simulink model "gm_sampleModel2076_4_sub"  (R2023a)
settings: Solver=VariableStepAuto  StartTime=0.0  StopTime=10.0  RelTol=1e-3
libraries: hdlsllib x2, simulink x1
settings Model: Creator=user1  LastModifiedBy=user1
settings OptimizationCC: BlockReduction=off  ConditionallyExecuteInputs=off
settings DebuggingCC: InheritedTsInSrcMsg=none

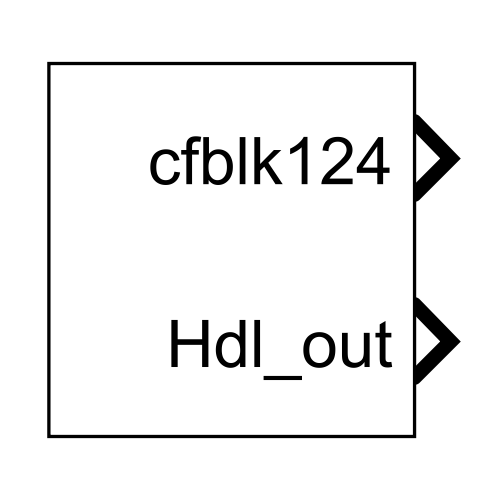
[thumbnail: Simulink's stored preview of the top-level diagram]
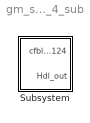
== system gm_sampleModel2076_4_sub ==
  Subsystem : Subsystem

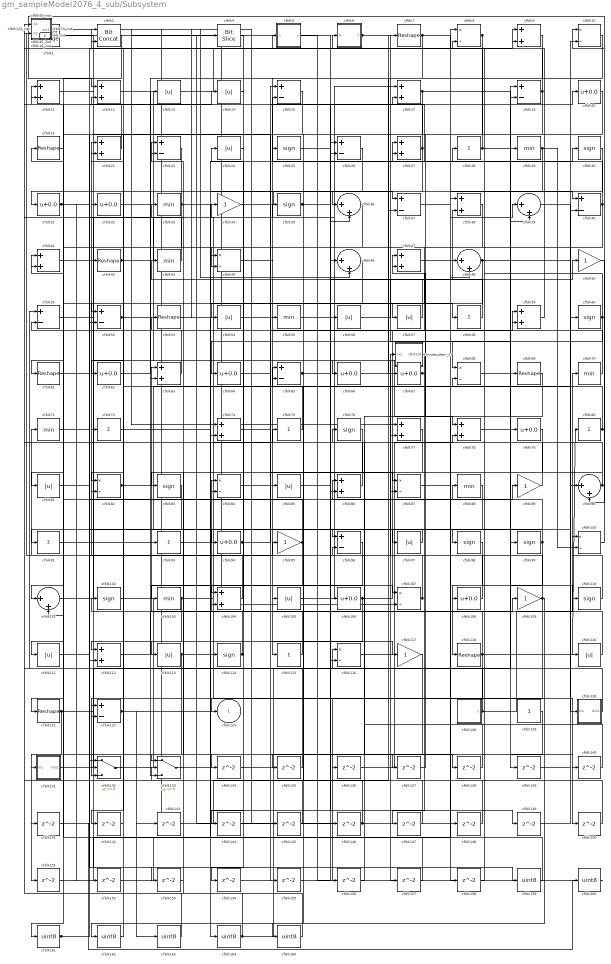
== system gm_sampleModel2076_4_sub/Subsystem ==
  Mysubsystem_27 : Subsystem
  cfblk1 : simulink/Logic and Bit Operations/Detect Change  vinit=0  OutDataTypeStr=uint8
      settings: LibrarySourceBlock=|
      | hdlsllib/Logic and Bit
      | Operations/Detect
      | Change
  cfblk{8,10,44,68,82,84,87,100,107,116} (10 alike) : Product  Inputs=*/  OutDataTypeStr=uint8  RndMeth=Zero  SaturateOnIntegerOverflow=on
  cfblk{36,39,46,48,90,101} (6 alike) : Sum  Inputs=|++  OutDataTypeStr=uint8
  cfblk{25,30,35,60,76,83,98..99,102,110,114} (11 alike) : Signum
  cfblk{29,33,43,55,70..71,88,103} (8 alike) : MinMax  OutDataTypeStr=uint8
  cfblk{9,11..12,17,22,27,38,41,47,59,63,74,77..78,86,104,112} (17 alike) : Sum  OutDataTypeStr=uint8
  cfblk{13..14,24,54,56..57,81,85,97,105,111,113,120} (13 alike) : Abs  OutDataTypeStr=uint8  SaturateOnIntegerOverflow=off
  cfblk{20,31..32,62,64,66..67,79,94,106,108} (11 alike) : Bias  Bias=0.0  SaturateOnIntegerOverflow=off
  cfblk{34,50,89,95,109,117} (6 alike) : Gain  OutDataTypeStr=uint8
  cfblk{28,58,72,75,80,91,93,115} (8 alike) : Sum  Inputs=+  OutDataTypeStr=uint8
  cfblk{7,21,42,53,61,69,118,121} (8 alike) : Reshape
  cfblk119_inst : Subsystem
  cfblk{15,19,23,26,37,40,51..52,65,96,122} (11 alike) : Sum  Inputs=+-  OutDataTypeStr=uint8
  cfblk123_inst : Subsystem
  cfblk128 : Subsystem  mask(Counter Limited){uplimit=double(7), tsamp=double(-1)}
      mask prompts: uplimit "Simulink:masks:UpperLimit_MP"; tsamp "Simulink:masks:SampleTime_MP"
      mask help: Simulink:masks:CounterLimited_MD
      mask init:
      | nbits = double(8);
      | tsamp = double(-1);
      | uplimit = double(7);
  cfblk129 : Constant  OutDataTypeStr=uint8  SampleTime=-1
  cfblk130 : Subsystem
  cfblk131 : Subsystem
  cfblk132 : Switch  OutDataTypeStr=uint8  SaturateOnIntegerOverflow=off  InputSameDT=off
  cfblk133 : Switch  OutDataTypeStr=uint8  SaturateOnIntegerOverflow=off  InputSameDT=off
  cfblk{134..158} (25 alike) : Delay  SampleTime=1
  cfblk{159..165} (7 alike) : DataTypeConversion  OutDataTypeStr=uint8  SaturateOnIntegerOverflow=off  RndMeth=Floor
  cfblk16_inst : Subsystem
  cfblk2 : hdlsllib/Logic and Bit Operations/Bit Concat  numInputs=2
  cfblk4 : hdlsllib/Logic and Bit Operations/Bit Slice  lidx=7  ridx=0
  cfblk45_inst : Subsystem
  cfblk5 : Subsystem  mask(Compare To Constant){relop=<=, const=double(3), OutDataTypeStr=uint8, ZeroCross=on}
      mask prompts: relop "Simulink:masks:Operator_MP"; const "Simulink:masks:ConstantValue_MP"; OutDataTypeStr "Simulink:masks:OutputDataType_MP"; ZeroCross "Simulink:masks:EnableZerocrossingDetection_MP"
      mask help: Simulink:masks:CompareToConstant_MD
      mask init:
      | OutDataTypeStr = 'uint8';
      | ZeroCross = 'on';
      | blkName = 'sampleModel2076_4_sub/Subsystem/cfblk5';
      | const = double(3);
      | const_str = '3.0';
      | const_val = double(3);
      | relop = '<=';
      | setValue = 'fixdt(0, 8)';
      | str = '<= 3';
      mask TypeOptions relop: == | ~= | < | <= | >= | >
      mask TypeOptions OutDataTypeStr: Simulink:masks:uint8 | Simulink:masks:boolean
      mask Callback ZeroCross: sl('zeroCrossEnable', gcbh);
      mask Display: disp(str)
  cfblk6 : Subsystem  mask(Detect Fall Nonpositive){vinit=double(0), InputProcessing=Elements as channels (sample based), OutDataTypeStr=uint8}
      mask prompts: vinit "Simulink:masks:InitialCondition_MP"; InputProcessing "Simulink:masks:InputProcessing_MP"; OutDataTypeStr "Simulink:masks:OutputDataType_MP"
      mask help: Simulink:masks:DetectFallNonpositive_MD
      mask init:
      | InputProcessing = 'Elements as channels (sample based)';
      | OutDataTypeStr = 'uint8';
      | vinit = double(0);
      mask TypeOptions InputProcessing: Simulink:masks:ColumnsAsChannelsFrameBased | Simulink:masks:ElementsAsChannelsSampleBased
      mask TypeOptions OutDataTypeStr: Simulink:masks:uint8 | Simulink:masks:boolean
      mask Display: fprintf('U <= 0\n&  NOT\nU/z <= 0')
  cfblk73_inst : Subsystem
  cfblk92_inst : Subsystem
  cfblk124 : Outport  OutDataTypeStr=uint8  SampleTime=1  VectorParamsAs1DForOutWhenUnconnected=off
  Hdl_out : Outport  Port=2  OutDataTypeStr=uint8  SampleTime=1
  wires:
  Mysubsystem_27/1(cfblk124) -> cfblk124/1
  cfblk1/1 -> cfblk159/1
  cfblk10/1 -> cfblk115/1
  cfblk100/1 -> cfblk12/1
  cfblk101/1 -> cfblk34/1
  cfblk102/1 -> cfblk116/1
  cfblk103/1 -> cfblk113/1, cfblk75/1
  cfblk104/1 -> cfblk71/1
  cfblk105/1 -> cfblk17/1
  cfblk106/1 -> cfblk59/1, cfblk112/1
  cfblk107/1 -> cfblk22/1, cfblk123_inst/2(in2)
  cfblk108/1 -> cfblk51/2
  cfblk109/1 -> cfblk162/1, cfblk156/1, Mysubsystem_27/1(In1)
  cfblk11/1 -> cfblk85/1
  cfblk110/1 -> cfblk70/1
  cfblk111/1 -> cfblk42/1
  cfblk112/1 -> cfblk109/1
  cfblk113/1 -> cfblk27/1, cfblk151/1, cfblk150/1
  cfblk114/1 -> cfblk102/1, cfblk84/1
  cfblk115/1 -> cfblk63/1
  cfblk116/1 -> cfblk88/1
  cfblk117/1 -> cfblk134/1
  cfblk118/1 -> cfblk24/1, cfblk132/3, cfblk80/1
  cfblk119_inst/1(out1) -> cfblk74/1
  cfblk12/1 -> cfblk114/1
  cfblk120/1 -> cfblk72/1
  cfblk121/1 -> cfblk79/1, cfblk141/1
  cfblk122/1 -> cfblk27/2, cfblk163/1, cfblk143/1
  cfblk123_inst/1(out1) -> cfblk77/1
  cfblk128/1(y) -> cfblk51/1, cfblk82/2, cfblk100/1
  cfblk129/1 -> cfblk131/1(In1)
  cfblk13/1 -> cfblk8/2
  cfblk130/1(Out1) -> cfblk33/1
  cfblk131/1(Out1) -> cfblk7/1
  cfblk132/1 -> cfblk69/1
  cfblk133/1 -> cfblk89/1
  cfblk134/1 -> cfblk19/2
  cfblk135/1 -> cfblk119_inst/2(in2)
  cfblk136/1 -> cfblk78/2
  cfblk137/1 -> cfblk47/1
  cfblk138/1 -> cfblk86/1
  cfblk139/1 -> cfblk90/1
  cfblk14/1 -> cfblk154/1
  cfblk140/1 -> cfblk8/1
  cfblk141/1 -> cfblk160/1
  cfblk142/1 -> cfblk22/2
  cfblk143/1 -> cfblk37/2
  cfblk144/1 -> cfblk39/2
  cfblk145/1 -> cfblk11/1
  cfblk146/1 -> cfblk23/1, Hdl_out/1
  cfblk147/1 -> cfblk101/2
  cfblk148/1 -> cfblk65/1
  cfblk149/1 -> cfblk40/2
  cfblk15/1 -> cfblk142/1
  cfblk150/1 -> cfblk92_inst/2(in2)
  cfblk151/1 -> cfblk74/2
  cfblk152/1 -> cfblk48/2
  cfblk153/1 -> cfblk133/2
  cfblk154/1 -> cfblk38/1
  cfblk155/1 -> cfblk46/1
  cfblk156/1 -> cfblk96/2
  cfblk157/1 -> cfblk21/1
  cfblk158/1 -> cfblk28/1
  cfblk159/1 -> cfblk32/1
  cfblk16_inst/1(out1) -> cfblk46/2
  cfblk160/1 -> cfblk1/1
  cfblk161/1 -> cfblk95/1, cfblk84/2
  cfblk162/1 -> cfblk2/1
  cfblk163/1 -> cfblk2/2
  cfblk164/1 -> cfblk26/2, cfblk16_inst/1(in1), cfblk106/1
  cfblk165/1 -> cfblk93/1
  cfblk17/1 -> cfblk81/1, cfblk29/1
  cfblk19/1 -> cfblk77/2, cfblk16_inst/2(in2), cfblk105/1
  cfblk2/1 -> cfblk161/1
  cfblk20/1 -> cfblk44/2
  cfblk21/1 -> cfblk111/1
  cfblk22/1 -> cfblk11/2
  cfblk23/1 -> cfblk62/1
  cfblk24/1 -> cfblk44/1
  cfblk25/1 -> cfblk87/1
  cfblk26/1 -> cfblk122/2
  cfblk27/1 -> cfblk45_inst/1(in1), cfblk144/1
  cfblk28/1 -> cfblk99/1, cfblk5/1(u)
  cfblk29/1 -> cfblk61/1, cfblk132/2, cfblk100/2
  cfblk30/1 -> cfblk52/1
  cfblk31/1 -> cfblk14/1, cfblk153/1, cfblk152/1
  cfblk32/1 -> cfblk97/1
  cfblk33/1 -> cfblk36/1, cfblk31/1, cfblk101/1, cfblk58/1
  cfblk34/1 -> cfblk37/1
  cfblk35/1 -> cfblk20/1, cfblk117/1
  cfblk36/1 -> cfblk63/2
  cfblk37/1 -> cfblk40/1
  cfblk38/1 -> cfblk54/1
  cfblk39/1 -> cfblk60/1
  cfblk4/1 -> cfblk94/1
  cfblk40/1 -> cfblk57/1, cfblk17/2, cfblk15/2
  cfblk41/1 -> cfblk6/1(U)
  cfblk42/1 -> cfblk66/1, cfblk30/1
  cfblk43/1 -> cfblk123_inst/1(in1)
  cfblk44/1 -> cfblk55/1
  cfblk45_inst/1(out1) -> cfblk4/1, cfblk148/1, cfblk145/1
  cfblk46/1 -> cfblk82/1
  cfblk47/1 -> cfblk38/2
  cfblk48/1 -> cfblk121/1, cfblk130/1(In1)
  cfblk5/1(y) -> cfblk36/2
  cfblk50/1 -> cfblk90/2
  cfblk51/1 -> cfblk158/1
  cfblk52/1 -> cfblk78/1, cfblk87/2
  cfblk53/1 -> cfblk146/1
  cfblk54/1 -> cfblk86/2
  cfblk55/1 -> cfblk135/1
  cfblk56/1 -> cfblk50/1
  cfblk57/1 -> cfblk43/1
  cfblk58/1 -> cfblk15/1
  cfblk59/1 -> cfblk9/1
  cfblk6/1(Y) -> cfblk68/1, cfblk139/1
  cfblk60/1 -> cfblk73_inst/2(in2), cfblk73_inst/1(in1), cfblk64/1
  cfblk61/1 -> cfblk132/1
  cfblk62/1 -> cfblk13/1
  cfblk63/1 -> cfblk41/1
  cfblk64/1 -> cfblk155/1
  cfblk65/1 -> cfblk26/1, cfblk149/1
  cfblk66/1 -> cfblk157/1
  cfblk67/1 -> cfblk53/1, cfblk147/1
  cfblk68/1 -> cfblk140/1
  cfblk69/1 -> cfblk136/1
  cfblk7/1 -> cfblk9/2, cfblk133/3
  cfblk70/1 -> cfblk47/2
  cfblk71/1 -> cfblk98/1
  cfblk72/1 -> cfblk25/1
  cfblk73_inst/1(out1) -> cfblk107/2
  cfblk74/1 -> cfblk19/1
  cfblk75/1 -> cfblk65/2
  cfblk76/1 -> cfblk165/1
  cfblk77/1 -> cfblk103/1
  cfblk78/1 -> cfblk110/1
  cfblk79/1 -> cfblk104/1
  cfblk8/1 -> cfblk52/2, cfblk45_inst/2(in2), cfblk112/2
  cfblk80/1 -> cfblk12/2, cfblk10/1
  cfblk81/1 -> cfblk35/1
  cfblk82/1 -> cfblk120/1, cfblk10/2
  cfblk83/1 -> cfblk122/1
  cfblk84/1 -> cfblk138/1
  cfblk85/1 -> cfblk48/1
  cfblk86/1 -> cfblk92_inst/1(in1)
  cfblk87/1 -> cfblk39/1
  cfblk88/1 -> cfblk137/1
  cfblk89/1 -> cfblk23/2
  cfblk9/1 -> cfblk67/1
  cfblk90/1 -> cfblk83/1, cfblk119_inst/1(in1)
  cfblk91/1 -> cfblk107/1
  cfblk92_inst/1(out1) -> cfblk56/1
  cfblk93/1 -> cfblk164/1
  cfblk94/1 -> cfblk59/2, cfblk116/2
  cfblk95/1 -> cfblk41/2, cfblk104/2
  cfblk96/1 -> cfblk133/1
  cfblk97/1 -> cfblk96/1
  cfblk98/1 -> cfblk118/1
  cfblk99/1 -> cfblk76/1, cfblk108/1, cfblk68/2, cfblk91/1

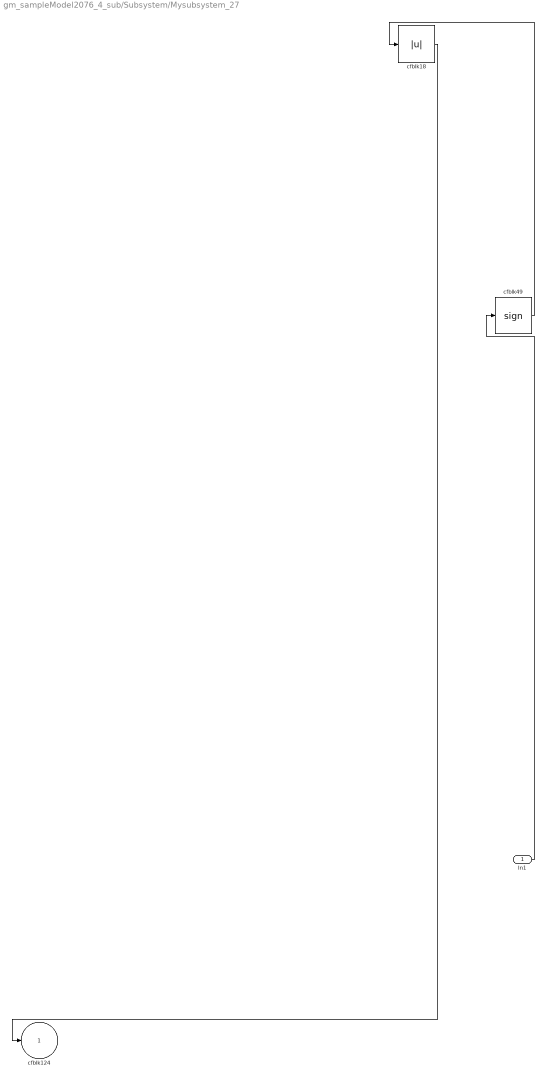
== system gm_sampleModel2076_4_sub/Subsystem/Mysubsystem_27 ==
  In1 : Inport  OutDataTypeStr=uint8  PortDimensions=1  SampleTime=1
  cfblk18 : Abs  SaturateOnIntegerOverflow=off
  cfblk49 : Signum
  cfblk124 : Outport  SampleTime=1  VectorParamsAs1DForOutWhenUnconnected=off
  wires:
  In1/1 -> cfblk49/1
  cfblk18/1 -> cfblk124/1
  cfblk49/1 -> cfblk18/1

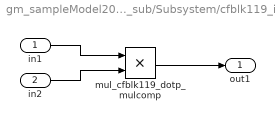
== system gm_sampleModel2076_4_sub/Subsystem/cfblk119_inst ==
  in1 : Inport  OutDataTypeStr=uint8  SampleTime=1
  in2 : Inport  Port=2  OutDataTypeStr=uint8  SampleTime=1
  mul_cfblk119_dotp_mulcomp : Product  Inputs=**  OutDataTypeStr=uint8  SampleTime=1
  out1 : Outport  OutDataTypeStr=uint8  SampleTime=1
  wires:
  in1/1 -> mul_cfblk119_dotp_mulcomp/1
  in2/1 -> mul_cfblk119_dotp_mulcomp/2
  mul_cfblk119_dotp_mulcomp/1 -> out1/1

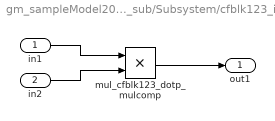
== system gm_sampleModel2076_4_sub/Subsystem/cfblk123_inst ==
  in1 : Inport  OutDataTypeStr=uint8  SampleTime=1
  in2 : Inport  Port=2  OutDataTypeStr=uint8  SampleTime=1
  mul_cfblk123_dotp_mulcomp : Product  Inputs=**  OutDataTypeStr=uint8  SampleTime=1
  out1 : Outport  OutDataTypeStr=uint8  SampleTime=1
  wires:
  in1/1 -> mul_cfblk123_dotp_mulcomp/1
  in2/1 -> mul_cfblk123_dotp_mulcomp/2
  mul_cfblk123_dotp_mulcomp/1 -> out1/1

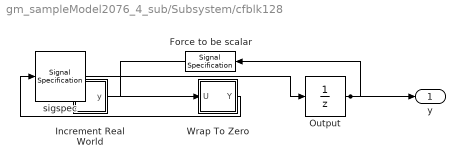
== system gm_sampleModel2076_4_sub/Subsystem/cfblk128 ==
  Force to be scalar : SignalSpecification  DisableCoverage=on  Dimensions=1
  Increment Real World : Subsystem  mask(Real World Value Increment){}
      mask help: Simulink:masks:RealWorldValueIncrement_MD
      mask Display: disp('V++')
  Output : UnitDelay  InitialCondition=0.0  SampleTime=tsamp  HasFrameUpgradeWarning=on
  Wrap To Zero : Subsystem  mask(Wrap To Zero){Threshold=double(7)}
      mask prompts: Threshold "Simulink:masks:Threshold_MP"
      mask help: Simulink:masks:WrapToZero_MD
  sigspec : SignalSpecification  OutDataTypeStr=uint8  Dimensions=1
  y : Outport  SampleTime=1
  wires:
  Force to be scalar/1 -> Increment Real World/1(u)
  Increment Real World/1(y) -> Wrap To Zero/1(U)
  Output/1 -> Force to be scalar/1, y/1
  Wrap To Zero/1(Y) -> sigspec/1
  sigspec/1 -> Output/1

== system gm_sampleModel2076_4_sub/Subsystem/cfblk130 ==
  In1 : Inport  OutDataTypeStr=uint8  PortDimensions=1  SampleTime=1
  Out1 : Outport  SampleTime=1
  wires:
  In1/1 -> Out1/1

== system gm_sampleModel2076_4_sub/Subsystem/cfblk131 ==
  In1 : Inport  OutDataTypeStr=uint8  PortDimensions=1  SampleTime=1
  Out1 : Outport  SampleTime=1
  wires:
  In1/1 -> Out1/1

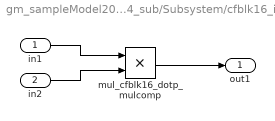
== system gm_sampleModel2076_4_sub/Subsystem/cfblk16_inst ==
  in1 : Inport  OutDataTypeStr=uint8  SampleTime=1
  in2 : Inport  Port=2  OutDataTypeStr=uint8  SampleTime=1
  mul_cfblk16_dotp_mulcomp : Product  Inputs=**  OutDataTypeStr=uint8  SampleTime=1
  out1 : Outport  OutDataTypeStr=uint8  SampleTime=1
  wires:
  in1/1 -> mul_cfblk16_dotp_mulcomp/1
  in2/1 -> mul_cfblk16_dotp_mulcomp/2
  mul_cfblk16_dotp_mulcomp/1 -> out1/1

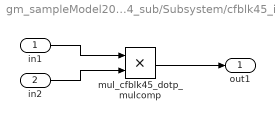
== system gm_sampleModel2076_4_sub/Subsystem/cfblk45_inst ==
  in1 : Inport  OutDataTypeStr=uint8  SampleTime=1
  in2 : Inport  Port=2  OutDataTypeStr=uint8  SampleTime=1
  mul_cfblk45_dotp_mulcomp : Product  Inputs=**  OutDataTypeStr=uint8  SampleTime=1
  out1 : Outport  OutDataTypeStr=uint8  SampleTime=1
  wires:
  in1/1 -> mul_cfblk45_dotp_mulcomp/1
  in2/1 -> mul_cfblk45_dotp_mulcomp/2
  mul_cfblk45_dotp_mulcomp/1 -> out1/1

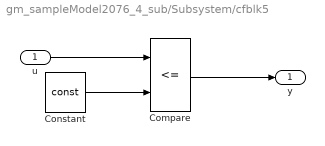
== system gm_sampleModel2076_4_sub/Subsystem/cfblk5 ==
  u : Inport  OutDataTypeStr=uint8  SampleTime=1
  Compare : RelationalOperator  Operator=<=  OutDataTypeStr=fixdt(0, 8)
  Constant : Constant  DisableCoverage=on  Value=const  OutDataTypeStr=Inherit: Inherit via back propagation  SampleTime=-1
  y : Outport  SampleTime=1
  wires:
  u/1 -> Compare/1
  Compare/1 -> y/1
  Constant/1 -> Compare/2

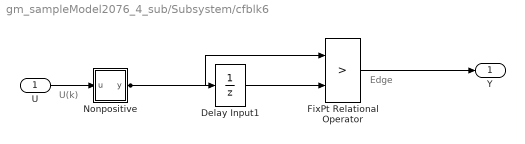
== system gm_sampleModel2076_4_sub/Subsystem/cfblk6 ==
  note: U(k)
  note: Edge
  U : Inport  OutDataTypeStr=uint8  SampleTime=1
  Delay Input1 : UnitDelay  Description=Store in Global RAM  DisableCoverage=on  InitialCondition=vinit  SampleTime=-1  HasFrameUpgradeWarning=on
  FixPt Relational Operator : RelationalOperator  Operator=>  OutDataTypeStr=fixdt(0, 8)  ZeroCross=off  InputSameDT=off
  Nonpositive : Subsystem  mask(Compare To Zero){relop=<=, OutDataTypeStr=boolean, ZeroCross=off}
      mask prompts: relop "Simulink:masks:Operator_MP"; OutDataTypeStr "Simulink:masks:OutputDataType_MP"; ZeroCross "Simulink:masks:EnableZerocrossingDetection_MP"
      mask help: Simulink:masks:CompareToZero_MD
      mask init:
      | OutDataTypeStr = 'boolean';
      | ZeroCross = 'off';
      | blkName = 'sampleModel2076_4_sub/Subsystem/cfblk6/Nonpositive';
      | relop = '<=';
      | setValue = 'boolean';
      mask TypeOptions relop: == | ~= | < | <= | >= | >
      mask TypeOptions OutDataTypeStr: Simulink:masks:uint8 | Simulink:masks:boolean
      mask Callback ZeroCross: sl('zeroCrossEnable', gcbh);
      mask Display: disp([relop,' 0'])
  Y : Outport  SampleTime=1
  wires:
  U/1 -> Nonpositive/1(u)
  Delay Input1/1 -> FixPt Relational Operator/2
  FixPt Relational Operator/1 -> Y/1
  Nonpositive/1(y) -> FixPt Relational Operator/1, Delay Input1/1

== system gm_sampleModel2076_4_sub/Subsystem/cfblk73_inst ==
  in1 : Inport  OutDataTypeStr=uint8  SampleTime=1
  in2 : Inport  Port=2  OutDataTypeStr=uint8  SampleTime=1
  mul_cfblk73_dotp_mulcomp : Product  Inputs=**  OutDataTypeStr=uint8  SampleTime=1
  out1 : Outport  OutDataTypeStr=uint8  SampleTime=1
  wires:
  in1/1 -> mul_cfblk73_dotp_mulcomp/1
  in2/1 -> mul_cfblk73_dotp_mulcomp/2
  mul_cfblk73_dotp_mulcomp/1 -> out1/1

== system gm_sampleModel2076_4_sub/Subsystem/cfblk92_inst ==
  in1 : Inport  OutDataTypeStr=uint8  SampleTime=1
  in2 : Inport  Port=2  OutDataTypeStr=uint8  SampleTime=1
  mul_cfblk92_dotp_mulcomp : Product  Inputs=**  OutDataTypeStr=uint8  SampleTime=1
  out1 : Outport  OutDataTypeStr=uint8  SampleTime=1
  wires:
  in1/1 -> mul_cfblk92_dotp_mulcomp/1
  in2/1 -> mul_cfblk92_dotp_mulcomp/2
  mul_cfblk92_dotp_mulcomp/1 -> out1/1

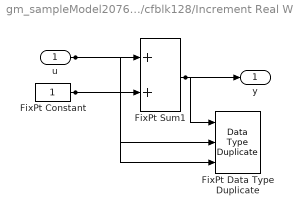
== system gm_sampleModel2076_4_sub/Subsystem/cfblk128/Increment Real World ==
  u : Inport  OutDataTypeStr=uint8  SampleTime=1
  FixPt Constant : Constant  DisableCoverage=on  OutDataTypeStr=Inherit: Inherit via back propagation  SampleTime=-1
  FixPt Data Type Duplicate : DataTypeDuplicate  DisableCoverage=on  NumInputPorts=3
  FixPt Sum1 : Sum  InputSameDT=on  OutDataTypeStr=Inherit: Inherit via back propagation  LockScale=on
  y : Outport  SampleTime=1
  wires:
  u/1 -> FixPt Sum1/1, FixPt Data Type Duplicate/2
  FixPt Constant/1 -> FixPt Sum1/2, FixPt Data Type Duplicate/3
  FixPt Sum1/1 -> FixPt Data Type Duplicate/1, y/1

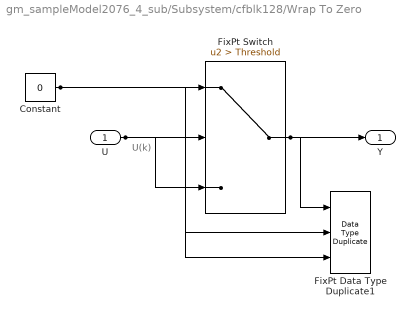
== system gm_sampleModel2076_4_sub/Subsystem/cfblk128/Wrap To Zero ==
  note: U(k)
  U : Inport  OutDataTypeStr=uint8  SampleTime=1
  Constant : Constant  DisableCoverage=on  Value=0  OutDataTypeStr=Inherit: Inherit via back propagation  SampleTime=-1
  FixPt Data Type Duplicate1 : DataTypeDuplicate  DisableCoverage=on  NumInputPorts=3
  FixPt Switch : Switch  Criteria=u2 > Threshold  Threshold=Threshold  OutDataTypeStr=Inherit: Inherit via back propagation  ZeroCross=off  SaturateOnIntegerOverflow=off  InputSameDT=off
  Y : Outport  SampleTime=1
  wires:
  U/1 -> FixPt Switch/3, FixPt Switch/2, FixPt Data Type Duplicate1/2
  Constant/1 -> FixPt Switch/1, FixPt Data Type Duplicate1/3
  FixPt Switch/1 -> FixPt Data Type Duplicate1/1, Y/1

== system gm_sampleModel2076_4_sub/Subsystem/cfblk6/Nonpositive ==
  u : Inport  OutDataTypeStr=uint8  SampleTime=1
  Compare : RelationalOperator  Operator=<=  OutDataTypeStr=boolean  ZeroCross=off
  Constant : Constant  DisableCoverage=on  Value=0  OutDataTypeStr=Inherit: Inherit via back propagation  SampleTime=-1  PreserveConstantTs=on
  y : Outport  SampleTime=1
  wires:
  u/1 -> Compare/1
  Compare/1 -> y/1
  Constant/1 -> Compare/2
